simulink model "Simulation_parfait"  (Simulink 6.0)
settings: Solver=ode3  StartTime=0.0  StopTime=10  FixedStep=5e-4  RelTol=5e-3
undefined symbols (not defined in the file or in its folder): sigbuilder_block
libraries: simulink x23, mblibv1 x15, aerolibtransform2 x5, vrlib x1
settings Model: LastModifiedBy=Yann
settings OptimizationCC: InlineInvariantSignals=off
settings SimMechanicsCC: VisDuringSimulation=on

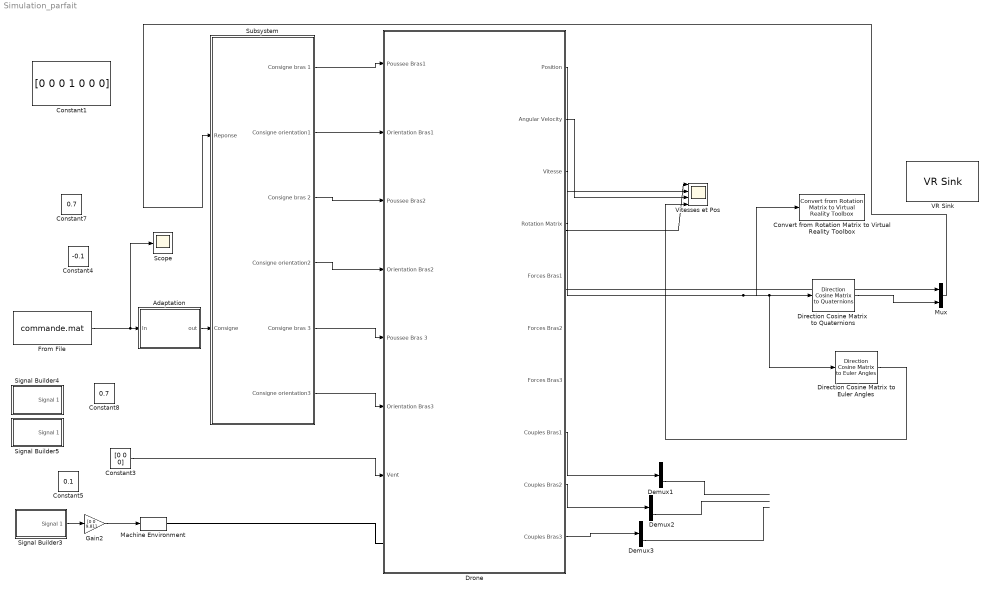
== system Simulation_parfait ==
  Adaptation : Subsystem
  Constant1 : Constant  Value=[0 0 0 1 0 0 0]
  Constant3 : Constant  Value=[0 0 0]
  Constant4 : Constant  Value=-0.1
  Constant5 : Constant  Value=0.1
  Constant7 : Constant  Value=0.7
  Constant8 : Constant  Value=0.7
  Convert from Rotation Matrix to Virtual Reality Toolbox : mblibv1/Utilities/Convert from Rotation Matrix to Virtual Reality Toolbox  Tag=Pose2VR
  Demux1 : Demux  Outputs=3
  Demux2 : Demux  Outputs=3
  Demux3 : Demux  Outputs=3
  Direction Cosine Matrix  to Quaternions : aerolibtransform2/Direction Cosine Matrix  to Quaternions
  Direction Cosine Matrix to Euler Angles : aerolibtransform2/Direction Cosine Matrix to Euler Angles
  Drone : Subsystem
  From File : FromFile  FileName=commande.mat  SampleTime=0
  Gain2 : Gain  Gain=[0 0 9.81]
  Machine Environment : mblibv1/Bodies/Machine Environment  Tag=Factory ground  DialogController=MECH.DialogSource  Opaque=on  PortType=env  PhysicalDomain=Mechanical  DialogTemplateClass=MECH.MachineEnvironment  SyncWhenCopied=off  Gravity=[0 0 9.81]  GravityUnits=m/s^2  GravityAsSignal=on  Dimensionality=Auto-detect  AnalysisType=Forward dynamics  LinearAssemblyTolerance=1e-3  LinearAssemblyToleranceUnits=m  AngularAssemblyTolerance=1e-3  AngularAssemblyToleranceUnits=rad  ConstraintSolverType=Stabilizing  ConstraintRelTolerance=1e-4  ConstraintAbsTolerance=1e-4  UseRobustSingularityHandling=off  StatePerturbationType=Fixed  PerturbationSize=1e-5  VisualizeMachine=on
  Mux : Mux  Inputs=2
  Scope : Scope
      settings: YMin=0  YMax=1  SaveName=ScopeData3
  Signal Builder3 : Subsystem  Tag=STV Subsys  LoadFcn=sigbuilder_block('load');  StartFcn=sigbuilder_block('start');  StopFcn=sigbuilder_block('stop');  ClipboardFcn=sigbuilder_block('clipboard');  mask(Sigbuilder block){}
      mask help: Sigbuilder GUI
      mask init:
      | if ~strcmp(get_param(bdroot(gcbh),'SimulationStatus'),'stopped') tuvar = sigbuilder_block('maskInit'); end
      settings: CopyFcn=sigbuilder_block('copy');  DeleteFcn=sigbuilder_block('delete');  ModelCloseFcn=sigbuilder_block('modelClose');  PreSaveFcn=sigbuilder_block('preSave');  NameChangeFcn=sigbuilder_block('namechange');  OpenFcn=sigbuilder_block('open',[39.75 63 664.5 410.25 ]);  CloseFcn=sigbuilder_block('close');
      mask Display: plot(0,0,100,100,[10,10,40,40,10],[80,20,20,80,80],[40,10],[50,50], [40,27,10],[65,72,56],[40,25,25,10],[28,28,43,43]);
  Signal Builder4 : Subsystem  Tag=STV Subsys  LoadFcn=sigbuilder_block('load');  StartFcn=sigbuilder_block('start');  StopFcn=sigbuilder_block('stop');  ClipboardFcn=sigbuilder_block('clipboard');  mask(Sigbuilder block){}
      mask help: Sigbuilder GUI
      mask init:
      | if ~strcmp(get_param(bdroot(gcbh),'SimulationStatus'),'stopped') tuvar = sigbuilder_block('maskInit'); end
      settings: CopyFcn=sigbuilder_block('copy');  DeleteFcn=sigbuilder_block('delete');  ModelCloseFcn=sigbuilder_block('modelClose');  PreSaveFcn=sigbuilder_block('preSave');  NameChangeFcn=sigbuilder_block('namechange');  OpenFcn=sigbuilder_block('open',[39.75 63 664.5 410.25 ]);  CloseFcn=sigbuilder_block('close');
      mask Display: plot(0,0,100,100,[10,10,40,40,10],[80,20,20,80,80],[40,10],[50,50], [40,27,10],[65,72,56],[40,25,25,10],[28,28,43,43]);
  Signal Builder5 : Subsystem  Tag=STV Subsys  LoadFcn=sigbuilder_block('load');  StartFcn=sigbuilder_block('start');  StopFcn=sigbuilder_block('stop');  ClipboardFcn=sigbuilder_block('clipboard');  mask(Sigbuilder block){}
      mask help: Sigbuilder GUI
      mask init:
      | if ~strcmp(get_param(bdroot(gcbh),'SimulationStatus'),'stopped') tuvar = sigbuilder_block('maskInit'); end
      settings: CopyFcn=sigbuilder_block('copy');  DeleteFcn=sigbuilder_block('delete');  ModelCloseFcn=sigbuilder_block('modelClose');  PreSaveFcn=sigbuilder_block('preSave');  NameChangeFcn=sigbuilder_block('namechange');  OpenFcn=sigbuilder_block('open',[75 91.5 664.5 410.25 ]);  CloseFcn=sigbuilder_block('close');
      mask Display: plot(0,0,100,100,[10,10,40,40,10],[80,20,20,80,80],[40,10],[50,50], [40,27,10],[65,72,56],[40,25,25,10],[28,28,43,43]);
  Subsystem : Subsystem
  VR Sink : vrlib/VR Sink  SampleTime=0.1  ViewEnable=on  RemoteChange=off  RemoteView=on  FieldsWritten=Drone.center.3.1.double#Drone.rotation.4.1.double  WorldFileName=drone2.WRL  AutoView=off  FigureProperties={}
  Vitesses et Pos : Scope  NumInputPorts=4
      settings: YMin=-0.15~-0.5~-9000~-5  YMax=0.25~0.9~4000~5  SaveName=ScopeData4
  wires:
  Drone/1(Position) -> Vitesses et Pos/1, Mux/1
  Drone/3(Vitesse) -> Vitesses et Pos/2
  Drone/2(Angular Velocity) -> Vitesses et Pos/3
  Drone/4(Rotation Matrix) -> Convert from Rotation Matrix to Virtual Reality Toolbox/1, Direction Cosine Matrix  to Quaternions/1, Direction Cosine Matrix to Euler Angles/1
  Constant3/1 -> Drone/7(Vent)
  Demux1/3 -> ?
  Demux2/3 -> ?
  Demux3/3 -> ?
  Drone/8(Couples Bras1) -> Demux1/1
  Drone/9(Couples Bras2) -> Demux2/1
  Drone/10(Couples Bras3) -> Demux3/1
  Signal Builder3/1(Signal 1) -> Gain2/1
  Gain2/1 -> Machine Environment/1
  Direction Cosine Matrix  to Quaternions/1 -> Mux/2
  Mux/1 -> Subsystem/1(Reponse)
  From File/1 -> Scope/1, Adaptation/1(In)
  Subsystem/1(Consigne bras 1) -> Drone/1(Poussee Bras1)
  Subsystem/5(Consigne bras 3) -> Drone/5(Poussee Bras 3)
  Subsystem/6(Consigne orientation3) -> Drone/6(Orientation Bras3)
  Direction Cosine Matrix to Euler Angles/1 -> Vitesses et Pos/4
  Subsystem/4(Consigne orientation2) -> Drone/4(Orientation Bras2)
  Subsystem/3(Consigne bras 2) -> Drone/3(Poussee Bras2)
  Subsystem/2(Consigne orientation1) -> Drone/2(Orientation Bras1)
  Adaptation/1(out) -> Subsystem/2(Consigne)
  connections:
  Drone/LConn1 -- Machine Environment/RConn1

== system Simulation_parfait/Adaptation ==
  In : Inport  Port=1  LatchInput=off
  Demux : Demux  Outputs=2
  Euler Angles to Quaternions : aerolibtransform2/Euler Angles to Quaternions
  Mux : Mux  Inputs=2
  Reshape : simulink/Math Operations/Reshape  OutputDimensionality=1-D array  OutputDimensions=[1,1]
  out : Outport
  wires:
  In/1 -> Demux/1
  Demux/2 -> Euler Angles to Quaternions/1
  Euler Angles to Quaternions/1 -> Mux/2
  Demux/1 -> Mux/1
  Mux/1 -> Reshape/1
  Reshape/1 -> out/1

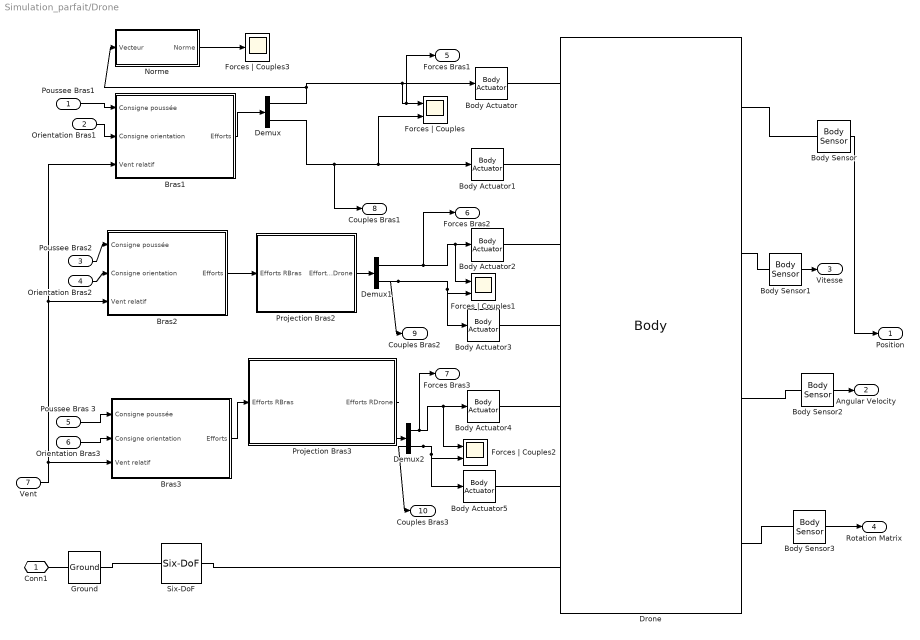
== system Simulation_parfait/Drone ==
  Poussee Bras1 : Inport  Port=1  LatchInput=off
  Orientation Bras1 : Inport  Port=2  LatchInput=off
  Poussee Bras2 : Inport  Port=3  LatchInput=off
  Orientation Bras2 : Inport  Port=4  LatchInput=off
  Poussee Bras 3 : Inport  Port=5  LatchInput=off
  Orientation Bras3 : Inport  Port=6  LatchInput=off
  Vent : Inport  Port=7  LatchInput=off
  Body Actuator : mblibv1/Sensors &  Actuators/Body Actuator  Opaque=on  PhysicalDomain=Mechanical  PortType=blob  ActuationStyle=Force  AngleUnits=deg  ArcVelocityUnits=deg/s  ArcAccelerationUnits=deg/s^2  CoordPositionUnits=m  VelocityUnits=m/s  AccelerationUnits=m/s^2  ForceUnits=N  TorqueUnits=N-m  ActiveIO=on  Width=3  DialogClass=MechanicalActuatorBlock  ReferenceFrame=Local (Body CS)  Angle=off  CoordPosition=on  Force=on  Torque=off
  Body Actuator1 : mblibv1/Sensors &  Actuators/Body Actuator  Opaque=on  PhysicalDomain=Mechanical  PortType=blob  ActuationStyle=Force  AngleUnits=deg  ArcVelocityUnits=deg/s  ArcAccelerationUnits=deg/s^2  CoordPositionUnits=m  VelocityUnits=m/s  AccelerationUnits=m/s^2  ForceUnits=N  TorqueUnits=N-m  ActiveIO=on  Width=3  DialogClass=MechanicalActuatorBlock  ReferenceFrame=Local (Body CS)  Angle=off  CoordPosition=on  Force=off  Torque=on
  Body Actuator2 : mblibv1/Sensors &  Actuators/Body Actuator  Opaque=on  PhysicalDomain=Mechanical  PortType=blob  ActuationStyle=Force  AngleUnits=deg  ArcVelocityUnits=deg/s  ArcAccelerationUnits=deg/s^2  CoordPositionUnits=m  VelocityUnits=m/s  AccelerationUnits=m/s^2  ForceUnits=N  TorqueUnits=N-m  ActiveIO=on  Width=3  DialogClass=MechanicalActuatorBlock  ReferenceFrame=Local (Body CS)  Angle=off  CoordPosition=on  Force=on  Torque=off
  Body Actuator3 : mblibv1/Sensors &  Actuators/Body Actuator  Opaque=on  PhysicalDomain=Mechanical  PortType=blob  ActuationStyle=Force  AngleUnits=deg  ArcVelocityUnits=deg/s  ArcAccelerationUnits=deg/s^2  CoordPositionUnits=m  VelocityUnits=m/s  AccelerationUnits=m/s^2  ForceUnits=N  TorqueUnits=N-m  ActiveIO=on  Width=3  DialogClass=MechanicalActuatorBlock  ReferenceFrame=Local (Body CS)  Angle=off  CoordPosition=on  Force=off  Torque=on
  Body Actuator4 : mblibv1/Sensors &  Actuators/Body Actuator  Opaque=on  PhysicalDomain=Mechanical  PortType=blob  ActuationStyle=Force  AngleUnits=deg  ArcVelocityUnits=deg/s  ArcAccelerationUnits=deg/s^2  CoordPositionUnits=m  VelocityUnits=m/s  AccelerationUnits=m/s^2  ForceUnits=N  TorqueUnits=N-m  ActiveIO=on  Width=3  DialogClass=MechanicalActuatorBlock  ReferenceFrame=Local (Body CS)  Angle=off  CoordPosition=on  Force=on  Torque=off
  Body Actuator5 : mblibv1/Sensors &  Actuators/Body Actuator  Opaque=on  PhysicalDomain=Mechanical  PortType=blob  ActuationStyle=Force  AngleUnits=deg  ArcVelocityUnits=deg/s  ArcAccelerationUnits=deg/s^2  CoordPositionUnits=m  VelocityUnits=m/s  AccelerationUnits=m/s^2  ForceUnits=N  TorqueUnits=N-m  ActiveIO=on  Width=3  DialogClass=MechanicalActuatorBlock  ReferenceFrame=Local (Body CS)  Angle=off  CoordPosition=on  Force=off  Torque=on
  Body Sensor : mblibv1/Sensors &  Actuators/Body Sensor  Opaque=on  PhysicalDomain=Mechanical  PortType=blob  Muxed=on  Pose=off  Angle=on  AngleUnits=deg  ArcVelocity=off  ArcVelocityUnits=deg/s  ArcAcceleration=off  ArcAccelerationUnits=deg/s^2  CoordPosition=on  CoordPositionUnits=m  Velocity=off  VelocityUnits=m/s  Acceleration=off  AccelerationUnits=m/s^2  Quaternion=on  QuaternionDT=off  QuaternionDDT=off  QuaternionUnits=off  OutputVector=[ 3 ]  ActiveIO=on  Width=3  DialogClass=MechanicalSensorBlock  ReferenceFrame=Absolute (World)
  Body Sensor1 : mblibv1/Sensors &  Actuators/Body Sensor  Opaque=on  PhysicalDomain=Mechanical  PortType=blob  Muxed=on  Pose=off  Angle=on  AngleUnits=deg  ArcVelocity=off  ArcVelocityUnits=deg/s  ArcAcceleration=off  ArcAccelerationUnits=deg/s^2  CoordPosition=off  CoordPositionUnits=m  Velocity=on  VelocityUnits=m/s  Acceleration=off  AccelerationUnits=m/s^2  Quaternion=on  QuaternionDT=off  QuaternionDDT=off  QuaternionUnits=off  OutputVector=[ 3 ]  ActiveIO=on  Width=3  DialogClass=MechanicalSensorBlock  ReferenceFrame=Absolute (World)
  Body Sensor2 : mblibv1/Sensors &  Actuators/Body Sensor  Opaque=on  PhysicalDomain=Mechanical  PortType=blob  Muxed=on  Pose=off  Angle=on  AngleUnits=deg  ArcVelocity=on  ArcVelocityUnits=deg/s  ArcAcceleration=off  ArcAccelerationUnits=deg/s^2  CoordPosition=off  CoordPositionUnits=m  Velocity=off  VelocityUnits=m/s  Acceleration=off  AccelerationUnits=m/s^2  Quaternion=on  QuaternionDT=off  QuaternionDDT=off  QuaternionUnits=off  OutputVector=[ 3 ]  ActiveIO=on  Width=3  DialogClass=MechanicalSensorBlock  ReferenceFrame=Absolute (World)
  Body Sensor3 : mblibv1/Sensors &  Actuators/Body Sensor  Opaque=on  PhysicalDomain=Mechanical  PortType=blob  Muxed=on  Pose=on  Angle=on  AngleUnits=deg  ArcVelocity=off  ArcVelocityUnits=deg/s  ArcAcceleration=off  ArcAccelerationUnits=deg/s^2  CoordPosition=off  CoordPositionUnits=m  Velocity=off  VelocityUnits=m/s  Acceleration=off  AccelerationUnits=m/s^2  Quaternion=on  QuaternionDT=off  QuaternionDDT=off  QuaternionUnits=off  OutputVector=[ 9 ]  ActiveIO=on  Width=9  DialogClass=MechanicalSensorBlock  ReferenceFrame=Absolute (World)
  Bras1 : Subsystem
  Bras2 : Subsystem
  Bras3 : Subsystem
  Demux : Demux  Outputs=2
  Demux1 : Demux  Outputs=2
  Demux2 : Demux  Outputs=2
  Drone : mblibv1/Bodies/Body  PhysicalDomain=mechanical  SubClassName=Unknown  LeftPortType=workingframe  RightPortType=workingframe  LConnTagsString=CS3|CS9|CS5|CS10|CS4|CS11|CS1  RConnTagsString=CS2|CS6|CS7|CS8  DialogClass=MechanicalBodyBlock  Mass=1.331  MassUnits=kg  InertiaUnits=kg*m^2  Inertia=[1e-2 9.762e-8 1.027e-6;9.762e-8 0.01 -6.855e-6; 1.027e-6 -6.855e-6 0.018 ]  Shape=Cylinder  ShapeDims=[1 1]  ShapeUnits=m  ShapeUse=false  Density=1  DensityUnits=kg/m^3  DensityUse=false  CG=Left$CG$[0 0 0]$WORLD$WORLD$m$[0 0 0]$Euler X-Y-Z$deg$WORLD$false  WorkingFrames=Right$CS2$[0 0 0]$CG$CG$m$[0 0 0]$Euler X-Y-Z$deg$WORLD$true#Left$CS3$[0.21 0 0]$CG$CG$m$[0 0 0]$Euler X-Y-Z$deg$WORLD$true#Left$CS9$[0.21 0 0]$CG$CG$m$[0 0 0]$Euler X-Y-Z$deg$WORLD$true#Left$CS5$[-0.105 0.1819 0]$CG$CG$m$[0 0 0]$Euler X-Y-Z$deg$WORLD$true#Left$CS10$[-0.105 0.1819 0]$CG$CG$m$[0 0 0]$Euler X-Y-Z$deg$WORLD$true#Left$CS4$[-0.105 -0.1819 0]$CG$CG$m$[0 0 0]$Euler X-Y-Z$deg$WORLD$true#Left$CS11$[-0.105 -0.1819 0]$CG$CG$m$[0 0 0]$Euler X-Y-Z$deg$WORLD$true#Right$CS6$[0 0 0]$CG$CG$m$[0 0 0]$Euler X-Y-Z$deg$WORLD$true#Right$CS7$[0 0 0]$CG$CG$m$[0 0 0]$Euler X-Y-Z$deg$WORLD$true#Right$CS8$[0 0 0]$CG$CG$m$[0 0 0]$Euler X-Y-Z$deg$WORLD$true#Left$CS1$[0 0 0]$CG$CG$m$[0 0 0]$Euler X-Y-Z$deg$WORLD$true#Right$CS12$[0 0 0]$CG$CG$m$[0 0 0]$Euler X-Y-Z$deg$WORLD$false
  Forces | Couples : Scope  NumInputPorts=2
      settings: YMin=-0.025~-1.5  YMax=0.04~0
  Forces | Couples1 : Scope  NumInputPorts=2
      settings: YMin=-4~-1.25  YMax=0.5~0
  Forces | Couples2 : Scope  NumInputPorts=2
      settings: YMin=-6~-1.5  YMax=1~1.25  SaveName=ScopeData2
  Forces | Couples3 : Scope
      settings: YMin=0  YMax=5.5  SaveName=ScopeData16
  Ground : mblibv1/Bodies/Ground  Opaque=on  LeftPortType=env  RightPortType=workingframe  PhysicalDomain=Mechanical  DialogClass=GroundBlock  CoordPosition=[0 0 0]  CoordPositionUnits=m  StateVectorMgrId=-1  MachineId=[1 0]  ShowEnvPort=on
  Norme : Subsystem  mask{ordre=2}
      mask Display: text(0.3,0.5,strcat('Norme',get_param(gcb, 'ordre')));
  Projection Bras2 : Subsystem
  Projection Bras3 : Subsystem
  Six-DoF : mblibv1/Joints/Six-DoF  PhysicalDomain=mechanical  SubClassName=Unknown  LeftPortType=blob  RightPortType=blob  LConnTagsString=__newl0  RConnTagsString=__newr0  NumSAPorts=0  CutJoint=off  MarkAsCut=off  Primitives=prismatic_prismatic_prismatic_spherical  PrimitiveProps=P1$INERTIAL$[1 0 0]$prismatic#P2$INERTIAL$[0 1 0]$prismatic#P3$INERTIAL$[0 0 1]$prismatic#S$INERTIAL$[0 0 0]$spherical  DialogClass=JointBlock
  Conn1 : PMIOPort  Port=1  Side=Left
  Position : Outport
  Angular Velocity : Outport  Port=2
  Vitesse : Outport  Port=3
  Rotation Matrix : Outport  Port=4
  Forces Bras1 : Outport  Port=5
  Forces Bras2 : Outport  Port=6
  Forces Bras3 : Outport  Port=7
  Couples Bras1 : Outport  Port=8
  Couples Bras2 : Outport  Port=9
  Couples Bras3 : Outport  Port=10
  wires:
  Body Sensor/1 -> Position/1
  Body Sensor2/1 -> Angular Velocity/1
  Body Sensor1/1 -> Vitesse/1
  Body Sensor3/1 -> Rotation Matrix/1
  Vent/1 -> Bras1/3(Vent relatif), Bras2/3(Vent relatif), Bras3/3(Vent relatif)
  Poussee Bras 3/1 -> Bras3/1(Consigne poussée)
  Orientation Bras2/1 -> Bras2/2(Consigne orientation)
  Orientation Bras3/1 -> Bras3/2(Consigne orientation)
  Orientation Bras1/1 -> Bras1/2(Consigne orientation)
  Poussee Bras1/1 -> Bras1/1(Consigne poussée)
  Poussee Bras2/1 -> Bras2/1(Consigne poussée)
  Demux1/1 -> Body Actuator2/1, Forces | Couples1/1, Forces Bras2/1
  Demux1/2 -> Body Actuator3/1, Forces | Couples1/2, Couples Bras2/1
  Projection Bras2/1(Efforts RDrone) -> Demux1/1
  Demux2/1 -> Body Actuator4/1, Forces | Couples2/1, Forces Bras3/1
  Demux2/2 -> Body Actuator5/1, Forces | Couples2/2, Couples Bras3/1
  Projection Bras3/1(Efforts RDrone) -> Demux2/1
  Bras1/1(Efforts) -> Demux/1
  Demux/1 -> Body Actuator/1, Forces | Couples/1, Forces Bras1/1, Norme/1(Vecteur)
  Demux/2 -> Body Actuator1/1, Forces | Couples/2, Couples Bras1/1
  Norme/1(Norme) -> Forces | Couples3/1
  Bras2/1(Efforts) -> Projection Bras2/1(Efforts RBras)
  Bras3/1(Efforts) -> Projection Bras3/1(Efforts RBras)
  connections:
  Body Actuator/RConn1 -- Drone/LConn1
  Body Actuator1/RConn1 -- Drone/LConn2
  Body Actuator2/RConn1 -- Drone/LConn3
  Body Actuator3/RConn1 -- Drone/LConn4
  Body Actuator4/RConn1 -- Drone/LConn5
  Body Actuator5/RConn1 -- Drone/LConn6
  Body Sensor/LConn1 -- Drone/RConn1
  Body Sensor1/LConn1 -- Drone/RConn2
  Drone/RConn3 -- Body Sensor2/LConn1
  Body Sensor3/LConn1 -- Drone/RConn4
  Six-DoF/RConn1 -- Drone/LConn7
  Ground/RConn1 -- Six-DoF/LConn1
  Conn1/RConn1 -- Ground/LConn1

== system Simulation_parfait/Signal Builder3 ==
  Demux : Demux  Tag=STV Demux  Outputs=1
  FromWs : FromWorkspace  Tag=STV FromWs  VariableName=tuvar  SampleTime=0  SigBuilderData=DataTag1  VnvData=DataTag2
      SigBuilderData=|
      | channels.label = 'Signal 1'
      | channels.allXData = {[0 10]}
      | channels.allYData = {[1 1]}
      | common.afterFinalStr = 'Extrapolate'
      | common.sampleTime = 0
      | dataSet.timeRange = [0 10]
      | dataSet.name = 'Group 1'
  Signal 1 : Outport  Tag=STV Outport
  wires:
  Demux/1 -> Signal 1/1
  FromWs/1 -> Demux/1

== system Simulation_parfait/Signal Builder4 ==
  Demux : Demux  Tag=STV Demux  Outputs=1
  FromWs : FromWorkspace  Tag=STV FromWs  VariableName=tuvar  SampleTime=0  SigBuilderData=DataTag3  VnvData=DataTag4
      SigBuilderData=|
      | channels.label = 'Signal 1'
      | channels.allXData = {[0 1.02 1.1 2.46 2.54 3.88 4.08 10]}
      | channels.allYData = {[0 0 1 1.005 0.005 0.0041018766756 0.805 0.8]}
      | common.afterFinalStr = 'Extrapolate'
      | common.sampleTime = 0
      | dataSet.timeRange = [0 10]
      | dataSet.name = 'Group 1'
  Signal 1 : Outport  Tag=STV Outport
  wires:
  Demux/1 -> Signal 1/1
  FromWs/1 -> Demux/1

== system Simulation_parfait/Signal Builder5 ==
  Demux : Demux  Tag=STV Demux  Outputs=1
  FromWs : FromWorkspace  Tag=STV FromWs  VariableName=tuvar  SampleTime=0  SigBuilderData=DataTag5  VnvData=DataTag6
      SigBuilderData=|
      | channels.label = 'Signal 1'
      | channels.allXData = {[0 5.92 6.1 7.4 7.78 8.78 8.94 10]}
      | channels.allYData = {[0 0 0.5 0.49 -0.4 -0.4 0 0]}
      | common.afterFinalStr = 'Extrapolate'
      | common.sampleTime = 0
      | dataSet.timeRange = [0 10]
      | dataSet.name = 'Group 1'
  Signal 1 : Outport  Tag=STV Outport
  wires:
  Demux/1 -> Signal 1/1
  FromWs/1 -> Demux/1

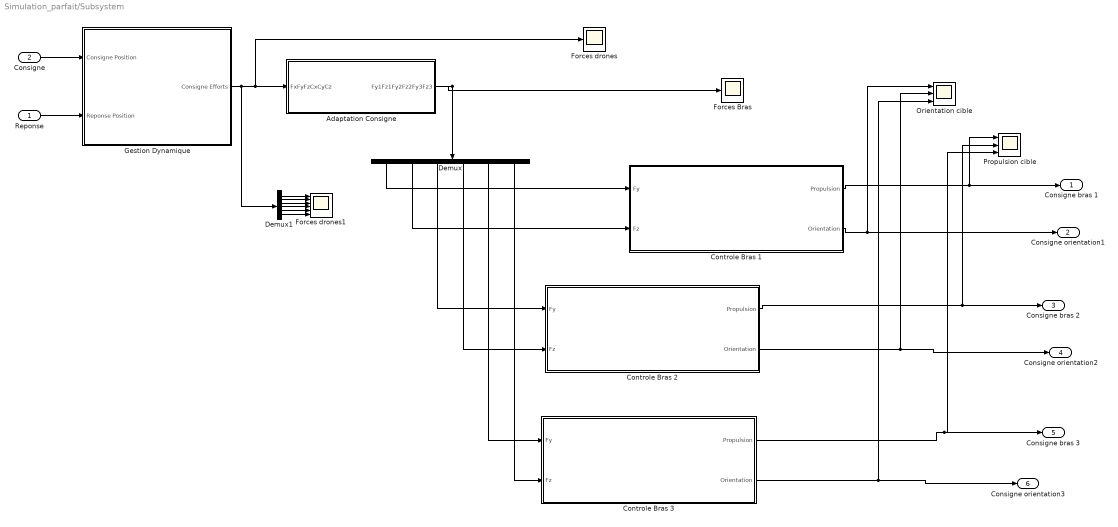
== system Simulation_parfait/Subsystem ==
  Reponse : Inport  Port=1  LatchInput=off
  Consigne : Inport  Port=2  LatchInput=off
  Adaptation Consigne : Subsystem  mask{l=0.21}
      mask prompts: l "Longueur Bras"
  Controle Bras 1 : Subsystem
  Controle Bras 2 : Subsystem
  Controle Bras 3 : Subsystem
  Demux : Demux  Orientation=down  Outputs=6
  Demux1 : Demux  Outputs=6
  Forces Bras : Scope
      settings: YMin=-0.24  YMax=2.77556e-017  SaveName=ScopeData14
  Forces drones : Scope
      settings: YMin=-0.01  YMax=0.0005  SaveName=ScopeData5
  Forces drones1 : Scope  NumInputPorts=6
      settings: YMin=-0.01~-5~-5~-5~-5~-5  YMax=0.0005~5~5~5~5~5  SaveName=ScopeData12
  Gestion Dynamique : Subsystem
  Orientation cible : Scope  NumInputPorts=3
      settings: YMin=-3.5~-5~-5  YMax=3.5~5~5  SaveName=ScopeData15
  Propulsion cible : Scope  NumInputPorts=3
      settings: YMin=1.9~0~-5  YMax=2.1~2~5  SaveName=ScopeData9
  Consigne bras 1 : Outport
  Consigne orientation1 : Outport  Port=2
  Consigne bras 2 : Outport  Port=3
  Consigne orientation2 : Outport  Port=4
  Consigne bras 3 : Outport  Port=5
  Consigne orientation3 : Outport  Port=6
  wires:
  Gestion Dynamique/1(Consigne Efforts) -> Adaptation Consigne/1(FxFyFzCxCyCz), Forces drones/1, Demux1/1
  Reponse/1 -> Gestion Dynamique/2(Reponse Position)
  Consigne/1 -> Gestion Dynamique/1(Consigne Position)
  Demux/1 -> Controle Bras 1/1(Fy)
  Demux/2 -> Controle Bras 1/2(Fz)
  Adaptation Consigne/1(Fy1Fz1Fy2Fz2Fy3Fz3) -> Demux/1, Forces Bras/1
  Demux/3 -> Controle Bras 2/1(Fy)
  Demux/4 -> Controle Bras 2/2(Fz)
  Demux/5 -> Controle Bras 3/1(Fy)
  Demux/6 -> Controle Bras 3/2(Fz)
  Controle Bras 1/1(Propulsion) -> Consigne bras 1/1, Propulsion cible/1
  Controle Bras 1/2(Orientation) -> Consigne orientation1/1, Orientation cible/1
  Controle Bras 2/1(Propulsion) -> Consigne bras 2/1, Propulsion cible/2
  Controle Bras 2/2(Orientation) -> Consigne orientation2/1, Orientation cible/2
  Controle Bras 3/1(Propulsion) -> Consigne bras 3/1, Propulsion cible/3
  Controle Bras 3/2(Orientation) -> Consigne orientation3/1, Orientation cible/3
  Demux1/1 -> Forces drones1/1
  Demux1/2 -> Forces drones1/2
  Demux1/3 -> Forces drones1/3
  Demux1/4 -> Forces drones1/4
  Demux1/5 -> Forces drones1/5
  Demux1/6 -> Forces drones1/6

== system Simulation_parfait/Drone/Bras1 ==
  Consigne poussée : Inport  Port=1  LatchInput=off
  Consigne orientation : Inport  Port=2  LatchInput=off
  Vent relatif : Inport  Port=3  LatchInput=off
  Bus Creator : BusCreator  DialogController=Simulink.DDGSource_Bus  Inputs=2
  Constant : Constant  Value=[0 0 0]
  Gain : Gain  Gain=pi
  Matrice rotation force : Subsystem
  Terminator : Terminator
  Efforts : Outport
  wires:
  Matrice rotation force/1(Force) -> Bus Creator/1  "Resultante"
  Constant/1 -> Bus Creator/2  "Moments"
  Bus Creator/1 -> Efforts/1
  Consigne orientation/1 -> Gain/1
  Consigne poussée/1 -> Matrice rotation force/1(Force poussée)
  Gain/1 -> Matrice rotation force/2(Angle orientation)
  Vent relatif/1 -> Terminator/1

== system Simulation_parfait/Drone/Bras2 ==
  Consigne poussée : Inport  Port=1  LatchInput=off
  Consigne orientation : Inport  Port=2  LatchInput=off
  Vent relatif : Inport  Port=3  LatchInput=off
  Bus Creator : BusCreator  DialogController=Simulink.DDGSource_Bus  Inputs=2
  Constant : Constant  Value=[0 0 0]
  Gain : Gain  Gain=pi
  Matrice rotation force : Subsystem
  Terminator : Terminator
  Efforts : Outport
  wires:
  Matrice rotation force/1(Force) -> Bus Creator/1  "Resultante"
  Constant/1 -> Bus Creator/2  "Moments"
  Bus Creator/1 -> Efforts/1
  Consigne orientation/1 -> Gain/1
  Consigne poussée/1 -> Matrice rotation force/1(Force poussée)
  Gain/1 -> Matrice rotation force/2(Angle orientation)
  Vent relatif/1 -> Terminator/1

== system Simulation_parfait/Drone/Bras3 ==
  Consigne poussée : Inport  Port=1  LatchInput=off
  Consigne orientation : Inport  Port=2  LatchInput=off
  Vent relatif : Inport  Port=3  LatchInput=off
  Bus Creator : BusCreator  DialogController=Simulink.DDGSource_Bus  Inputs=2
  Constant : Constant  Value=[0 0 0]
  Gain : Gain  Gain=pi
  Matrice rotation force : Subsystem
  Terminator : Terminator
  Efforts : Outport
  wires:
  Matrice rotation force/1(Force) -> Bus Creator/1  "Resultante"
  Constant/1 -> Bus Creator/2  "Moments"
  Bus Creator/1 -> Efforts/1
  Consigne orientation/1 -> Gain/1
  Consigne poussée/1 -> Matrice rotation force/1(Force poussée)
  Gain/1 -> Matrice rotation force/2(Angle orientation)
  Vent relatif/1 -> Terminator/1

== system Simulation_parfait/Drone/Norme ==
  Vecteur : Inport  Port=1  LatchInput=off
  Constant1 : Constant  Value=ordre
  Math Function : Math  Operator=pow  SaturateOnIntegerOverflow=on
  Math Function1 : Math  Operator=reciprocal  SaturateOnIntegerOverflow=on
  Math Function2 : Math  Operator=pow  SaturateOnIntegerOverflow=on
  Sum of Elements : Sum  Inputs=+  OutScaling=2^-10
  Norme : Outport
  wires:
  Math Function/1 -> Sum of Elements/1
  Vecteur/1 -> Math Function/1
  Constant1/1 -> Math Function/2, Math Function1/1
  Math Function1/1 -> Math Function2/2
  Sum of Elements/1 -> Math Function2/1
  Math Function2/1 -> Norme/1

== system Simulation_parfait/Drone/Projection Bras2 ==
  note: Forces
  note: Moments
  Efforts RBras : Inport  Port=1  LatchInput=off
  Bus Creator : BusCreator  DialogController=Simulink.DDGSource_Bus  Inputs=2
  Demux : Demux  Outputs=2
  Gain : Gain  Gain=[cos(2*pi/3) -sin(2*pi/3) 0 ; sin(2*pi/3) cos(2*pi/3) 0; 0 0 1]  Multiplication=Matrix(K*u) (u vector)
  Gain1 : Gain  Gain=[cos(2*pi/3) -sin(2*pi/3) 0 ; sin(2*pi/3) cos(2*pi/3) 0; 0 0 1]  Multiplication=Matrix(K*u) (u vector)
  Efforts RDrone : Outport
  wires:
  Efforts RBras/1 -> Demux/1
  Demux/1 -> Gain/1
  Demux/2 -> Gain1/1
  Bus Creator/1 -> Efforts RDrone/1
  Gain/1 -> Bus Creator/1
  Gain1/1 -> Bus Creator/2

== system Simulation_parfait/Drone/Projection Bras3 ==
  note: Forces
  note: Moments
  Efforts RBras : Inport  Port=1  LatchInput=off
  Bus Creator : BusCreator  DialogController=Simulink.DDGSource_Bus  Inputs=2
  Demux : Demux  Outputs=2
  Matrice de Rotation : Gain  Gain=[cos(4*pi/3) -sin(4*pi/3) 0 ; sin(4*pi/3) cos(4*pi/3) 0; 0 0 1]  Multiplication=Matrix(K*u) (u vector)
  "Matrice de rotation " : Gain  Gain=[cos(4*pi/3) -sin(4*pi/3) 0 ; sin(4*pi/3) cos(4*pi/3) 0; 0 0 1]  Multiplication=Matrix(K*u) (u vector)
  Efforts RDrone : Outport
  wires:
  Efforts RBras/1 -> Demux/1
  Demux/1 -> Matrice de Rotation/1
  Demux/2 -> "Matrice de rotation "/1
  Bus Creator/1 -> Efforts RDrone/1
  Matrice de Rotation/1 -> Bus Creator/1
  "Matrice de rotation "/1 -> Bus Creator/2

== system Simulation_parfait/Subsystem/Adaptation Consigne ==
  FxFyFzCxCyCz : Inport  Port=1  LatchInput=off
  Matrice Correction : Constant  Value=[1 1 1 1/l 1/l -1/l]
  Matrice Transformation : Constant  Value=(1/3)*[0 2 0 0 0 1; 0 0 1 0 2 0; -sqrt(3) -1 0 0 0 1; 0 0 1 -sqrt(3) -1 0; sqrt(3) -1 0 0 0 1; 0 0 1 sqrt(3) -1 0]  VectorParams1D=off
  Product : Product  Multiplication=Matrix(*)  RndMeth=Zero
  Product1 : Product  RndMeth=Zero
  Fy1Fz1Fy2Fz2Fy3Fz3 : Outport
  wires:
  Product/1 -> Fy1Fz1Fy2Fz2Fy3Fz3/1
  Matrice Transformation/1 -> Product/1
  Matrice Correction/1 -> Product1/2
  FxFyFzCxCyCz/1 -> Product1/1
  Product1/1 -> Product/2

== system Simulation_parfait/Subsystem/Controle Bras 1 ==
  Fy : Inport  Port=1  LatchInput=off
  Fz : Inport  Port=2  LatchInput=off
  Adaptation Consigne1 : Subsystem  mask{a=2e-5, b=1e-3, c=2e-3}
  Controle Bras1 : Subsystem
  Gain : Gain  Gain=60/(500*2*pi)
  Gain5 : Gain  Gain=1/pi
  Propulsion : Outport
  Orientation : Outport  Port=2
  wires:
  Controle Bras1/1(Force Propulsion) -> Adaptation Consigne1/1(Force)
  Adaptation Consigne1/1(Consigne Omega) -> Gain/1
  Gain/1 -> Propulsion/1
  Fy/1 -> Controle Bras1/1(Fyc)
  Fz/1 -> Controle Bras1/2(Fzc)
  Gain5/1 -> Orientation/1
  Controle Bras1/2(Angle Orientation) -> Gain5/1

== system Simulation_parfait/Subsystem/Controle Bras 2 ==
  Fy : Inport  Port=1  LatchInput=off
  Fz : Inport  Port=2  LatchInput=off
  Adaptation Consigne1 : Subsystem  mask{a=2e-5, b=1e-3, c=2e-3}
  Controle Bras1 : Subsystem
  Gain : Gain  Gain=60/(500*2*pi)
  Gain5 : Gain  Gain=1/pi
  Propulsion : Outport
  Orientation : Outport  Port=2
  wires:
  Controle Bras1/1(Force Propulsion) -> Adaptation Consigne1/1(Force)
  Adaptation Consigne1/1(Consigne Omega) -> Gain/1
  Gain/1 -> Propulsion/1
  Fy/1 -> Controle Bras1/1(Fyc)
  Fz/1 -> Controle Bras1/2(Fzc)
  Gain5/1 -> Orientation/1
  Controle Bras1/2(Angle Orientation) -> Gain5/1

== system Simulation_parfait/Subsystem/Controle Bras 3 ==
  Fy : Inport  Port=1  LatchInput=off
  Fz : Inport  Port=2  LatchInput=off
  Adaptation Consigne1 : Subsystem  mask{a=2e-5, b=1e-3, c=2e-3}
  Controle Bras1 : Subsystem
  Gain : Gain  Gain=60/(500*2*pi)
  Gain5 : Gain  Gain=1/pi
  Propulsion : Outport
  Orientation : Outport  Port=2
  wires:
  Controle Bras1/1(Force Propulsion) -> Adaptation Consigne1/1(Force)
  Adaptation Consigne1/1(Consigne Omega) -> Gain/1
  Gain/1 -> Propulsion/1
  Fy/1 -> Controle Bras1/1(Fyc)
  Fz/1 -> Controle Bras1/2(Fzc)
  Gain5/1 -> Orientation/1
  Controle Bras1/2(Angle Orientation) -> Gain5/1

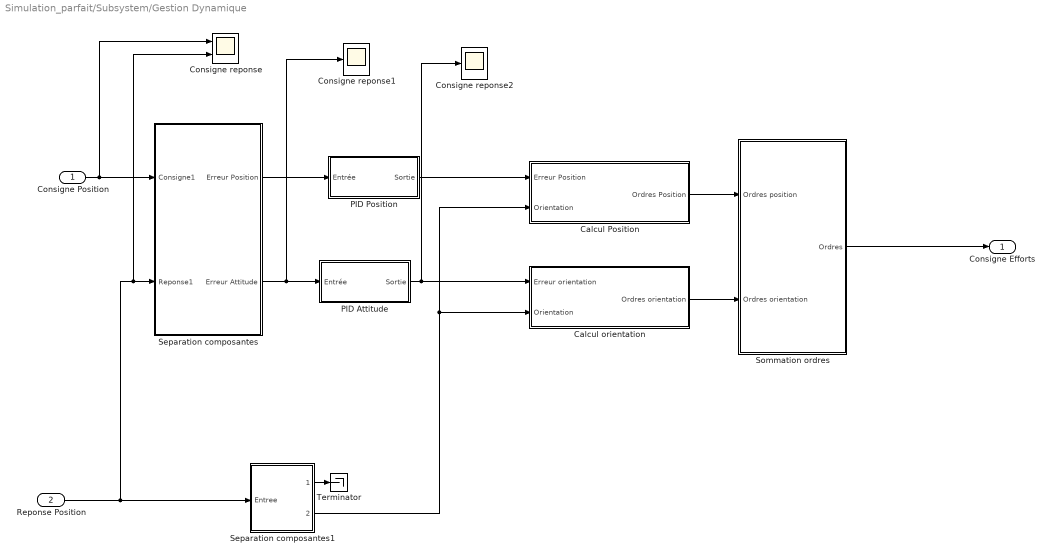
== system Simulation_parfait/Subsystem/Gestion Dynamique ==
  Consigne Position : Inport  Port=1  LatchInput=off
  Reponse Position : Inport  Port=2  LatchInput=off
  Calcul Position : Subsystem
  Calcul orientation : Subsystem
  Consigne reponse : Scope  NumInputPorts=2
      settings: YMin=0~-0.05  YMax=1~1.1  SaveName=ScopeData6
  Consigne reponse1 : Scope
      settings: YMin=0  YMax=1  SaveName=ScopeData8
  Consigne reponse2 : Scope
      settings: YMin=0  YMax=1  SaveName=ScopeData13
  PID Attitude : Subsystem  mask{kp=0.3, ki=0.1, kd=1, kdd=0}
  PID Position : Subsystem  mask{kp=100, ki=4, kd=1, kdd=0}
  Separation composantes : Subsystem
  Separation composantes1 : Subsystem
  Sommation ordres : Subsystem
  Terminator : Terminator
  Consigne Efforts : Outport
  wires:
  Reponse Position/1 -> Separation composantes1/1(Entree), Separation composantes/2(Reponse1), Consigne reponse/2
  Separation composantes1/2(Orientation) -> Calcul Position/2(Orientation), Calcul orientation/2(Orientation)
  Sommation ordres/1(Ordres) -> Consigne Efforts/1
  Separation composantes1/1(Position) -> Terminator/1
  PID Position/1(Sortie) -> Calcul Position/1(Erreur Position)
  Calcul Position/1(Ordres Position) -> Sommation ordres/1(Ordres position)
  Calcul orientation/1(Ordres orientation) -> Sommation ordres/2(Ordres orientation)
  PID Attitude/1(Sortie) -> Calcul orientation/1(Erreur orientation), Consigne reponse2/1
  Consigne Position/1 -> Separation composantes/1(Consigne1), Consigne reponse/1
  Separation composantes/1(Erreur Position) -> PID Position/1(Entrée)
  Separation composantes/2(Erreur Attitude) -> PID Attitude/1(Entrée), Consigne reponse1/1

== system Simulation_parfait/Drone/Bras1/Matrice rotation force ==
  Force poussée : Inport  Port=1  LatchInput=off
  Angle orientation : Inport  Port=2  LatchInput=off
  Constant : Constant  Value=0
  Cos : Trigonometry  Operator=cos
  Gain : Gain  Gain=[ 1 1 -1 ]
  Mux : Mux  Inputs=3
  Product : Product  RndMeth=Zero
  Reshape : simulink/Math Operations/Reshape  OutputDimensionality=1-D array  OutputDimensions=[1,1]
  Sin : Trigonometry
  Force : Outport
  wires:
  Angle orientation/1 -> Cos/1, Sin/1
  Constant/1 -> Mux/1
  Cos/1 -> Mux/3
  Sin/1 -> Mux/2
  Mux/1 -> Reshape/1
  Gain/1 -> Product/1
  Force poussée/1 -> Product/2
  Product/1 -> Force/1
  Reshape/1 -> Gain/1

== system Simulation_parfait/Drone/Bras2/Matrice rotation force ==
  Force poussée : Inport  Port=1  LatchInput=off
  Angle orientation : Inport  Port=2  LatchInput=off
  Constant : Constant  Value=0
  Cos : Trigonometry  Operator=cos
  Gain : Gain  Gain=[ 1 1 -1 ]
  Mux : Mux  Inputs=3
  Product : Product  RndMeth=Zero
  Reshape : simulink/Math Operations/Reshape  OutputDimensionality=1-D array  OutputDimensions=[1,1]
  Sin : Trigonometry
  Force : Outport
  wires:
  Angle orientation/1 -> Cos/1, Sin/1
  Constant/1 -> Mux/1
  Cos/1 -> Mux/3
  Sin/1 -> Mux/2
  Mux/1 -> Reshape/1
  Gain/1 -> Product/1
  Force poussée/1 -> Product/2
  Product/1 -> Force/1
  Reshape/1 -> Gain/1

== system Simulation_parfait/Drone/Bras3/Matrice rotation force ==
  Force poussée : Inport  Port=1  LatchInput=off
  Angle orientation : Inport  Port=2  LatchInput=off
  Constant : Constant  Value=0
  Cos : Trigonometry  Operator=cos
  Gain : Gain  Gain=[ 1 1 -1 ]
  Mux : Mux  Inputs=3
  Product : Product  RndMeth=Zero
  Reshape : simulink/Math Operations/Reshape  OutputDimensionality=1-D array  OutputDimensions=[1,1]
  Sin : Trigonometry
  Force : Outport
  wires:
  Angle orientation/1 -> Cos/1, Sin/1
  Constant/1 -> Mux/1
  Cos/1 -> Mux/3
  Sin/1 -> Mux/2
  Mux/1 -> Reshape/1
  Gain/1 -> Product/1
  Force poussée/1 -> Product/2
  Product/1 -> Force/1
  Reshape/1 -> Gain/1

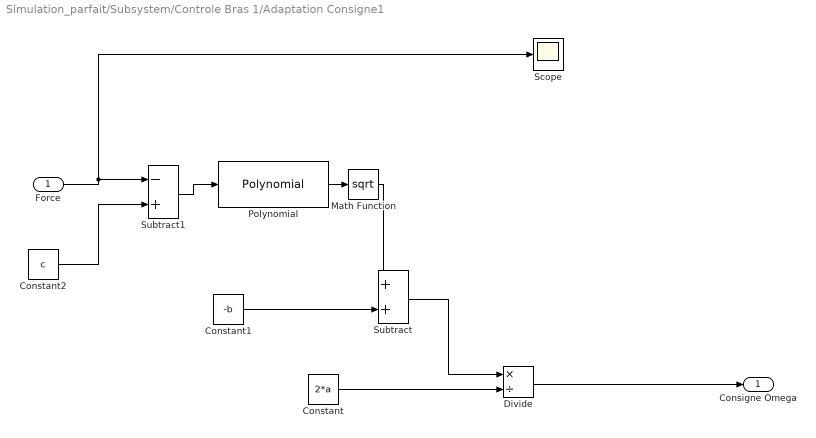
== system Simulation_parfait/Subsystem/Controle Bras 1/Adaptation Consigne1 ==
  Force : Inport  Port=1  LatchInput=off
  Constant : Constant  Value=2*a
  Constant1 : Constant  Value=-b
  Constant2 : Constant  Value=c
  Divide : Product  Inputs=*/  OutScaling=2^-10
  Math Function : Math  Operator=sqrt  SaturateOnIntegerOverflow=on
  Polynomial : simulink/Math Operations/Polynomial  coefs=[-4*a b*b]
  Scope : Scope
      settings: YMin=0  YMax=1000  SaveName=ScopeData7
  Subtract : Sum  OutScaling=2^-10
  Subtract1 : Sum  Inputs=-+  OutScaling=2^-10
  Consigne Omega : Outport
  wires:
  Constant/1 -> Divide/2
  Constant1/1 -> Subtract/2
  Subtract/1 -> Divide/1
  Divide/1 -> Consigne Omega/1
  Math Function/1 -> Subtract/1
  Polynomial/1 -> Math Function/1
  Force/1 -> Scope/1, Subtract1/1
  Subtract1/1 -> Polynomial/1
  Constant2/1 -> Subtract1/2

== system Simulation_parfait/Subsystem/Controle Bras 1/Controle Bras1 ==
  Fyc : Inport  Port=1  LatchInput=off
  Fzc : Inport  Port=2  LatchInput=off
  Complex to Magnitude-Angle : ComplexToMagnitudeAngle
  Real-Imag to Complex : RealImagToComplex
  Unary Minus : simulink/Math Operations/Unary Minus  DoSatur=off
  Force Propulsion : Outport
  Angle Orientation : Outport  Port=2
  wires:
  Real-Imag to Complex/1 -> Complex to Magnitude-Angle/1
  Complex to Magnitude-Angle/2 -> Angle Orientation/1
  Complex to Magnitude-Angle/1 -> Force Propulsion/1
  Fyc/1 -> Real-Imag to Complex/2
  Fzc/1 -> Unary Minus/1
  Unary Minus/1 -> Real-Imag to Complex/1

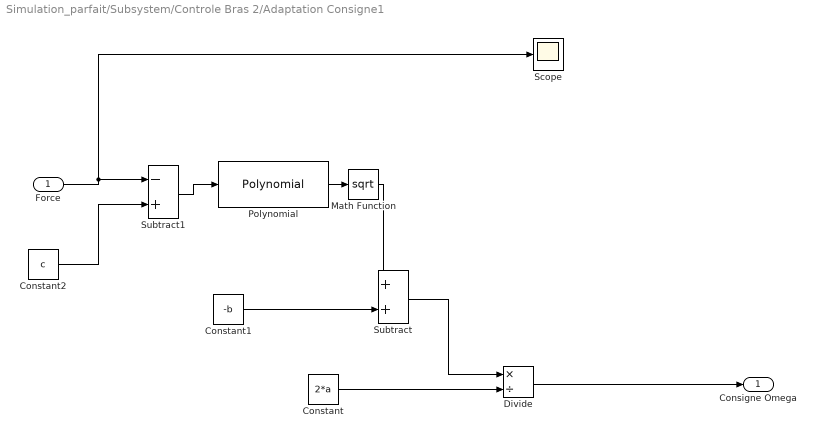
== system Simulation_parfait/Subsystem/Controle Bras 2/Adaptation Consigne1 ==
  Force : Inport  Port=1  LatchInput=off
  Constant : Constant  Value=2*a
  Constant1 : Constant  Value=-b
  Constant2 : Constant  Value=c
  Divide : Product  Inputs=*/  OutScaling=2^-10
  Math Function : Math  Operator=sqrt  SaturateOnIntegerOverflow=on
  Polynomial : simulink/Math Operations/Polynomial  coefs=[-4*a b*b]
  Scope : Scope
      settings: YMin=0  YMax=1000  SaveName=ScopeData7
  Subtract : Sum  OutScaling=2^-10
  Subtract1 : Sum  Inputs=-+  OutScaling=2^-10
  Consigne Omega : Outport
  wires:
  Constant/1 -> Divide/2
  Constant1/1 -> Subtract/2
  Subtract/1 -> Divide/1
  Divide/1 -> Consigne Omega/1
  Math Function/1 -> Subtract/1
  Polynomial/1 -> Math Function/1
  Force/1 -> Scope/1, Subtract1/1
  Subtract1/1 -> Polynomial/1
  Constant2/1 -> Subtract1/2

== system Simulation_parfait/Subsystem/Controle Bras 2/Controle Bras1 ==
  Fyc : Inport  Port=1  LatchInput=off
  Fzc : Inport  Port=2  LatchInput=off
  Complex to Magnitude-Angle : ComplexToMagnitudeAngle
  Real-Imag to Complex : RealImagToComplex
  Unary Minus : simulink/Math Operations/Unary Minus  DoSatur=off
  Force Propulsion : Outport
  Angle Orientation : Outport  Port=2
  wires:
  Real-Imag to Complex/1 -> Complex to Magnitude-Angle/1
  Complex to Magnitude-Angle/2 -> Angle Orientation/1
  Complex to Magnitude-Angle/1 -> Force Propulsion/1
  Fyc/1 -> Real-Imag to Complex/2
  Fzc/1 -> Unary Minus/1
  Unary Minus/1 -> Real-Imag to Complex/1

== system Simulation_parfait/Subsystem/Controle Bras 3/Adaptation Consigne1 ==
  Force : Inport  Port=1  LatchInput=off
  Constant : Constant  Value=2*a
  Constant1 : Constant  Value=-b
  Constant2 : Constant  Value=c
  Divide : Product  Inputs=*/  OutScaling=2^-10
  Math Function : Math  Operator=sqrt  SaturateOnIntegerOverflow=on
  Polynomial : simulink/Math Operations/Polynomial  coefs=[-4*a b*b]
  Scope : Scope
      settings: YMin=0  YMax=1000  SaveName=ScopeData7
  Subtract : Sum  OutScaling=2^-10
  Subtract1 : Sum  Inputs=-+  OutScaling=2^-10
  Consigne Omega : Outport
  wires:
  Constant/1 -> Divide/2
  Constant1/1 -> Subtract/2
  Subtract/1 -> Divide/1
  Divide/1 -> Consigne Omega/1
  Math Function/1 -> Subtract/1
  Polynomial/1 -> Math Function/1
  Force/1 -> Scope/1, Subtract1/1
  Subtract1/1 -> Polynomial/1
  Constant2/1 -> Subtract1/2

== system Simulation_parfait/Subsystem/Controle Bras 3/Controle Bras1 ==
  Fyc : Inport  Port=1  LatchInput=off
  Fzc : Inport  Port=2  LatchInput=off
  Complex to Magnitude-Angle : ComplexToMagnitudeAngle
  Real-Imag to Complex : RealImagToComplex
  Unary Minus : simulink/Math Operations/Unary Minus  DoSatur=off
  Force Propulsion : Outport
  Angle Orientation : Outport  Port=2
  wires:
  Real-Imag to Complex/1 -> Complex to Magnitude-Angle/1
  Complex to Magnitude-Angle/2 -> Angle Orientation/1
  Complex to Magnitude-Angle/1 -> Force Propulsion/1
  Fyc/1 -> Real-Imag to Complex/2
  Fzc/1 -> Unary Minus/1
  Unary Minus/1 -> Real-Imag to Complex/1

== system Simulation_parfait/Subsystem/Gestion Dynamique/Calcul Position ==
  Erreur Position : Inport  Port=1  LatchInput=off
  Orientation : Inport  Port=2  LatchInput=off
  Constant : Constant  Value=0
  Constant1 : Constant  Value=0
  Constant2 : Constant  Value=0
  Demux : Demux  Outputs=3
  Mux : Mux  Inputs=6
  Product : Product  Multiplication=Matrix(*)  RndMeth=Zero
  Quaternions to  Direction Cosine Matrix : aerolibtransform2/Quaternions to  Direction Cosine Matrix
  Reshape5 : simulink/Math Operations/Reshape  OutputDimensionality=1-D array  OutputDimensions=[1,1]
  Ordres Position : Outport
      settings: BusObject=perturbations
  wires:
  Mux/1 -> Reshape5/1
  Reshape5/1 -> Ordres Position/1
  Product/1 -> Demux/1
  Demux/1 -> Mux/1
  Demux/2 -> Mux/2
  Demux/3 -> Mux/3
  Constant2/1 -> Mux/6
  Constant1/1 -> Mux/5
  Constant/1 -> Mux/4
  Quaternions to  Direction Cosine Matrix/1 -> Product/1
  Orientation/1 -> Quaternions to  Direction Cosine Matrix/1
  Erreur Position/1 -> Product/2

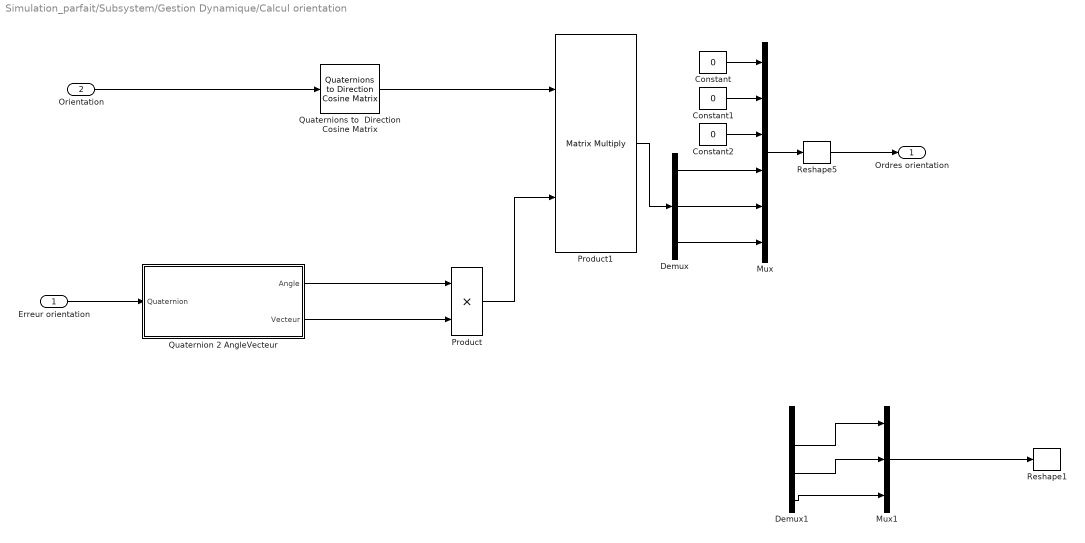
== system Simulation_parfait/Subsystem/Gestion Dynamique/Calcul orientation ==
  Erreur orientation : Inport  Port=1  LatchInput=off
  Orientation : Inport  Port=2  LatchInput=off
  Constant : Constant  Value=0
  Constant1 : Constant  Value=0
  Constant2 : Constant  Value=0
  Demux : Demux  Outputs=3
  Demux1 : Demux
  Mux : Mux  Inputs=6
  Mux1 : Mux  Inputs=3
  Product : Product  RndMeth=Zero
  Product1 : Product  Multiplication=Matrix(*)  RndMeth=Zero
  Quaternion 2 AngleVecteur : Subsystem
  Quaternions to  Direction Cosine Matrix : aerolibtransform2/Quaternions to  Direction Cosine Matrix
  Reshape1 : simulink/Math Operations/Reshape  OutputDimensionality=1-D array  OutputDimensions=[1,1]
  Reshape5 : simulink/Math Operations/Reshape  OutputDimensionality=1-D array  OutputDimensions=[1,1]
  Ordres orientation : Outport
      settings: BusObject=perturbations
  wires:
  Mux/1 -> Reshape5/1
  Reshape5/1 -> Ordres orientation/1
  Constant/1 -> Mux/1
  Constant1/1 -> Mux/2
  Constant2/1 -> Mux/3
  Demux/1 -> Mux/4
  Demux/2 -> Mux/5
  Demux/3 -> Mux/6
  Product1/1 -> Demux/1
  Orientation/1 -> Quaternions to  Direction Cosine Matrix/1
  Quaternion 2 AngleVecteur/2(Vecteur) -> Product/2
  Quaternion 2 AngleVecteur/1(Angle) -> Product/1
  Erreur orientation/1 -> Quaternion 2 AngleVecteur/1(Quaternion)
  Quaternions to  Direction Cosine Matrix/1 -> Product1/1
  Mux1/1 -> Reshape1/1
  Demux1/4 -> Mux1/3
  Demux1/3 -> Mux1/2
  Demux1/2 -> Mux1/1
  Product/1 -> Product1/2

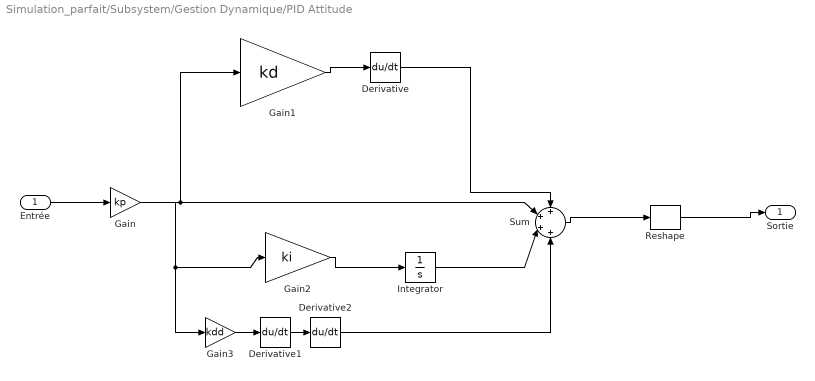
== system Simulation_parfait/Subsystem/Gestion Dynamique/PID Attitude ==
  Entrée : Inport  Port=1  LatchInput=off
  Derivative : Derivative
  Derivative1 : Derivative
  Derivative2 : Derivative
  Gain : Gain  Gain=kp
  Gain1 : Gain  Gain=kd
  Gain2 : Gain  Gain=ki
  Gain3 : Gain  Gain=kdd
  Integrator : Integrator
  Reshape : simulink/Math Operations/Reshape  OutputDimensionality=1-D array  OutputDimensions=[1,1]
  Sum : Sum  Inputs=++++
  Sortie : Outport
      settings: BusObject=perturbations
  wires:
  Entrée/1 -> Gain/1
  Gain/1 -> Sum/2, Gain1/1, Gain2/1, Gain3/1
  Derivative/1 -> Sum/1
  Integrator/1 -> Sum/3
  Gain2/1 -> Integrator/1
  Gain1/1 -> Derivative/1
  Sum/1 -> Reshape/1
  Gain3/1 -> Derivative1/1
  Derivative1/1 -> Derivative2/1
  Derivative2/1 -> Sum/4
  Reshape/1 -> Sortie/1

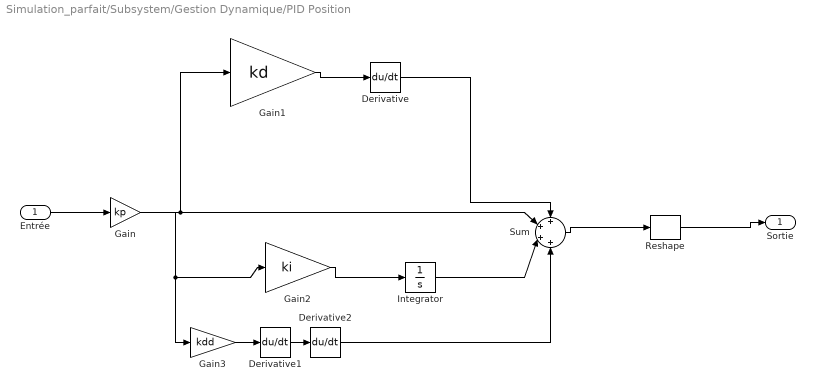
== system Simulation_parfait/Subsystem/Gestion Dynamique/PID Position ==
  Entrée : Inport  Port=1  LatchInput=off
  Derivative : Derivative
  Derivative1 : Derivative
  Derivative2 : Derivative
  Gain : Gain  Gain=kp
  Gain1 : Gain  Gain=kd
  Gain2 : Gain  Gain=ki
  Gain3 : Gain  Gain=kdd
  Integrator : Integrator
  Reshape : simulink/Math Operations/Reshape  OutputDimensionality=1-D array  OutputDimensions=[1,1]
  Sum : Sum  Inputs=++++
  Sortie : Outport
      settings: BusObject=perturbations
  wires:
  Entrée/1 -> Gain/1
  Gain/1 -> Sum/2, Gain1/1, Gain2/1, Gain3/1
  Derivative/1 -> Sum/1
  Integrator/1 -> Sum/3
  Gain2/1 -> Integrator/1
  Gain1/1 -> Derivative/1
  Sum/1 -> Reshape/1
  Gain3/1 -> Derivative1/1
  Derivative1/1 -> Derivative2/1
  Derivative2/1 -> Sum/4
  Reshape/1 -> Sortie/1

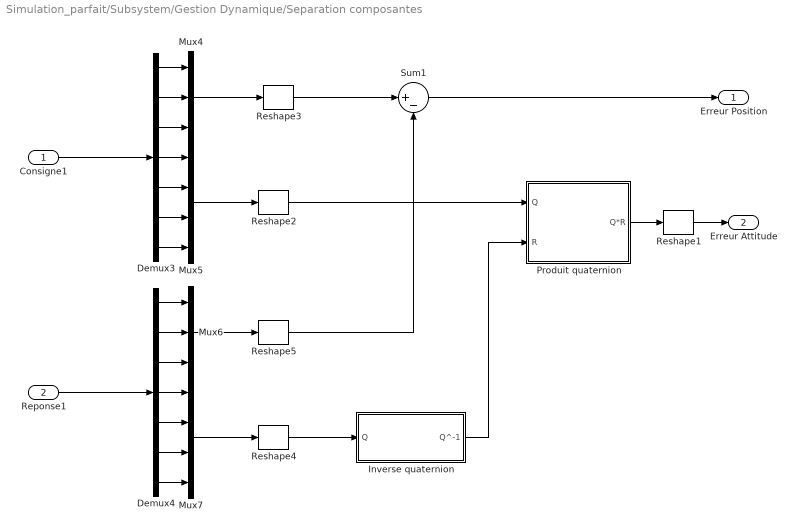
== system Simulation_parfait/Subsystem/Gestion Dynamique/Separation composantes ==
  Consigne1 : Inport  Port=1  LatchInput=off
  Reponse1 : Inport  Port=2  LatchInput=off
  Demux3 : Demux  Outputs=7
  Demux4 : Demux  Outputs=7
  Inverse quaternion : Subsystem
  Mux4 : Mux  Inputs=3
  Mux5 : Mux
  Mux6 : Mux  Inputs=3
  Mux7 : Mux
  Produit quaternion : Subsystem
  Reshape{1..5} (5 alike) : simulink/Math Operations/Reshape  OutputDimensionality=1-D array  OutputDimensions=[1,1]
  Sum1 : Sum  Inputs=|+-
  Erreur Position : Outport
      settings: BusObject=perturbations
  Erreur Attitude : Outport  Port=2
      settings: BusObject=perturbations
  wires:
  Consigne1/1 -> Demux3/1
  Demux3/4 -> Mux5/1
  Demux3/5 -> Mux5/2
  Demux3/6 -> Mux5/3
  Demux3/7 -> Mux5/4
  Demux3/3 -> Mux4/3
  Demux3/2 -> Mux4/2
  Demux3/1 -> Mux4/1
  Mux5/1 -> Reshape2/1
  Mux4/1 -> Reshape3/1
  Demux4/4 -> Mux7/1
  Demux4/5 -> Mux7/2
  Demux4/6 -> Mux7/3
  Demux4/7 -> Mux7/4
  Demux4/3 -> Mux6/3
  Demux4/2 -> Mux6/2
  Demux4/1 -> Mux6/1
  Reponse1/1 -> Demux4/1
  Mux7/1 -> Reshape4/1
  Mux6/1 -> Reshape5/1
  Reshape3/1 -> Sum1/1
  Reshape5/1 -> Sum1/2
  Sum1/1 -> Erreur Position/1
  Reshape4/1 -> Inverse quaternion/1(Q)
  Reshape2/1 -> Produit quaternion/1(Q)
  Inverse quaternion/1(Q^-1) -> Produit quaternion/2(R)
  Produit quaternion/1(Q*R) -> Reshape1/1
  Reshape1/1 -> Erreur Attitude/1

== system Simulation_parfait/Subsystem/Gestion Dynamique/Separation composantes1 ==
  Entree : Inport  Port=1  LatchInput=off
  Demux1 : Demux  Outputs=7
  Mux : Mux  Inputs=3
  Mux1 : Mux
  Reshape : simulink/Math Operations/Reshape  OutputDimensionality=1-D array  OutputDimensions=[1,1]
  Reshape1 : simulink/Math Operations/Reshape  OutputDimensionality=1-D array  OutputDimensions=[1,1]
  Position : Outport
      settings: BusObject=perturbations
  Orientation : Outport  Port=2
      settings: BusObject=perturbations
  wires:
  Entree/1 -> Demux1/1
  Demux1/4 -> Mux1/1
  Demux1/5 -> Mux1/2
  Demux1/6 -> Mux1/3
  Demux1/7 -> Mux1/4
  Demux1/3 -> Mux/3
  Demux1/2 -> Mux/2
  Demux1/1 -> Mux/1
  Mux1/1 -> Reshape/1
  Mux/1 -> Reshape1/1
  Reshape/1 -> Orientation/1
  Reshape1/1 -> Position/1

== system Simulation_parfait/Subsystem/Gestion Dynamique/Sommation ordres ==
  Ordres position : Inport  Port=1  LatchInput=off
  Ordres orientation : Inport  Port=2  LatchInput=off
  Sum : Sum
  Ordres : Outport
      settings: BusObject=perturbations
  wires:
  Ordres orientation/1 -> Sum/2
  Sum/1 -> Ordres/1
  Ordres position/1 -> Sum/1

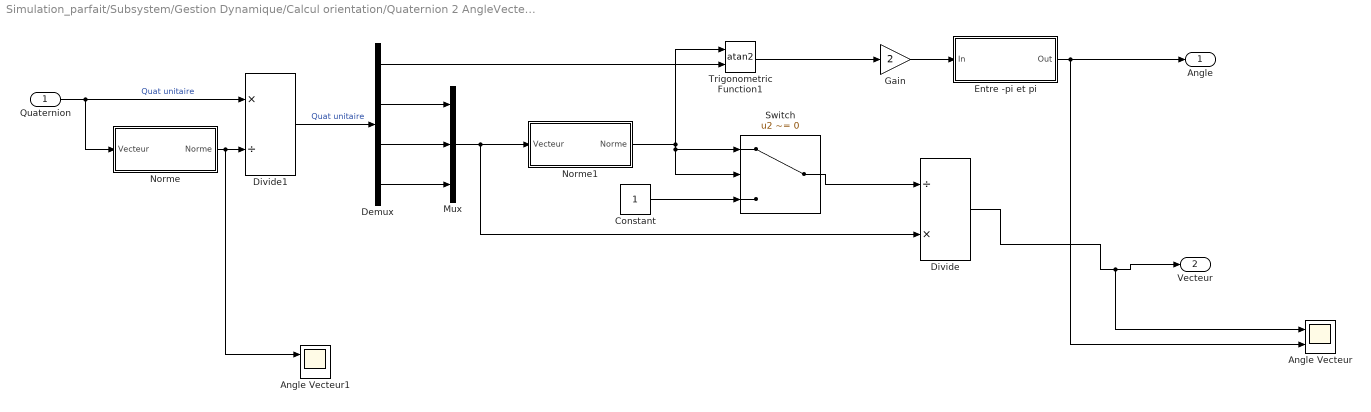
== system Simulation_parfait/Subsystem/Gestion Dynamique/Calcul orientation/Quaternion 2 AngleVecteur ==
  Quaternion : Inport  Port=1  LatchInput=off
  Angle Vecteur : Scope  NumInputPorts=2
      settings: YMin=-5~-5  YMax=5~5  SaveName=ScopeData10
  Angle Vecteur1 : Scope  NumInputPorts=2
      settings: YMin=0.007~-5  YMax=0.01025~5  SaveName=ScopeData17
  Constant : Constant
  Demux : Demux
  Divide : Product  Inputs=/*  OutScaling=2^-10
  Divide1 : Product  Inputs=*/  OutScaling=2^-10
  Entre -pi et pi : Subsystem  mask{ordre=2}
  Gain : Gain  Gain=2
  Mux : Mux  Inputs=3
  Norme : Subsystem  mask{ordre=2}
      mask Display: text(0.3,0.5,strcat('Norme',get_param(gcb, 'ordre')));
  Norme1 : Subsystem  mask{ordre=2}
      mask Display: text(0.3,0.5,strcat('Norme',get_param(gcb, 'ordre')));
  Switch : Switch  Criteria=u2 ~= 0
  Trigonometric Function1 : Trigonometry  Operator=atan2
  Angle : Outport
  Vecteur : Outport  Port=2
  wires:
  Quaternion/1 -> Divide1/1, Norme/1(Vecteur)  "Quat unitaire"
  Trigonometric Function1/1 -> Gain/1
  Mux/1 -> Norme1/1(Vecteur), Divide/2
  Demux/2 -> Mux/1
  Demux/3 -> Mux/2
  Demux/4 -> Mux/3
  Norme1/1(Norme) -> Trigonometric Function1/1, Switch/2, Switch/1
  Demux/1 -> Trigonometric Function1/2
  Switch/1 -> Divide/1
  Constant/1 -> Switch/3
  Entre -pi et pi/1(Out) -> Angle/1, Angle Vecteur/2
  Gain/1 -> Entre -pi et pi/1(In)
  Divide/1 -> Vecteur/1, Angle Vecteur/1
  Divide1/1 -> Demux/1  "Quat unitaire"
  Norme/1(Norme) -> Divide1/2, Angle Vecteur1/1

== system Simulation_parfait/Subsystem/Gestion Dynamique/Separation composantes/Inverse quaternion ==
  Q : Inport  Port=1  LatchInput=off
  Gain : Gain  Gain=[1 -1 -1 -1]
  Q^-1 : Outport
  wires:
  Q/1 -> Gain/1
  Gain/1 -> Q^-1/1

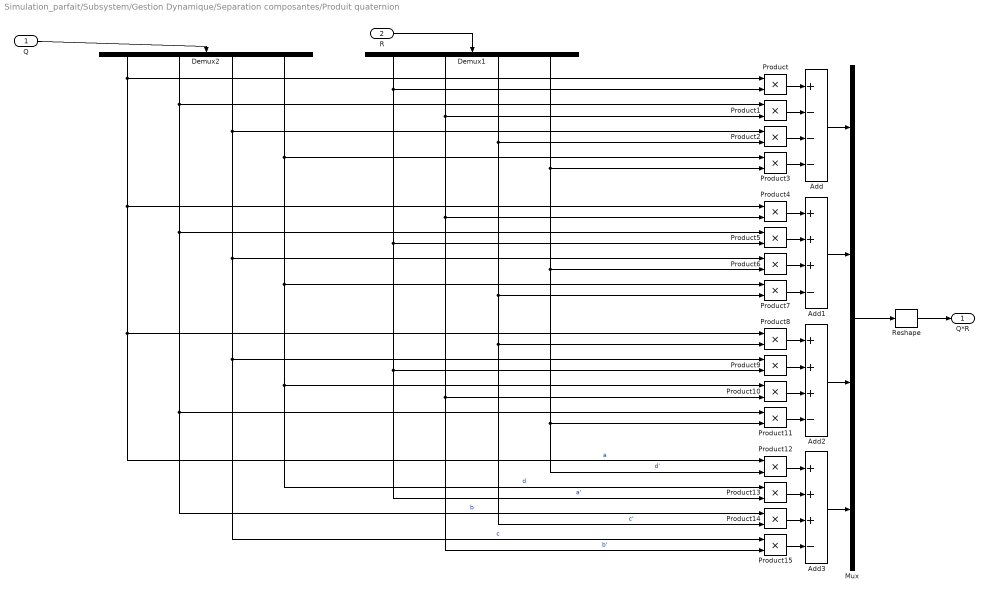
== system Simulation_parfait/Subsystem/Gestion Dynamique/Separation composantes/Produit quaternion ==
  Q : Inport  Port=1  LatchInput=off
  R : Inport  Port=2  LatchInput=off
  Add : Sum  Inputs=+---  OutScaling=2^-10
  Add1 : Sum  Inputs=+++-  OutScaling=2^-10
  Add2 : Sum  Inputs=+++-  OutScaling=2^-10
  Add3 : Sum  Inputs=+++-  OutScaling=2^-10
  Demux1 : Demux  Orientation=down
  Demux2 : Demux  Orientation=down
  Mux : Mux
  Product{,1..15} (16 alike) : Product  RndMeth=Zero
  Reshape : simulink/Math Operations/Reshape  OutputDimensionality=1-D array  OutputDimensions=[1,1]
  Q*R : Outport
  wires:
  R/1 -> Demux1/1
  Q/1 -> Demux2/1
  Mux/1 -> Reshape/1
  Reshape/1 -> Q*R/1
  Demux2/1 -> Product/1, Product4/1, Product8/1, Product12/1  "a"
  Add/1 -> Mux/1
  Add1/1 -> Mux/2
  Add2/1 -> Mux/3
  Add3/1 -> Mux/4
  Product3/1 -> Add/4
  Product2/1 -> Add/3
  Product1/1 -> Add/2
  Product/1 -> Add/1
  Product7/1 -> Add1/4
  Product6/1 -> Add1/3
  Product5/1 -> Add1/2
  Product4/1 -> Add1/1
  Product11/1 -> Add2/4
  Product10/1 -> Add2/3
  Product9/1 -> Add2/2
  Product8/1 -> Add2/1
  Product15/1 -> Add3/4
  Product14/1 -> Add3/3
  Product13/1 -> Add3/2
  Product12/1 -> Add3/1
  Demux2/2 -> Product1/1, Product5/1, Product11/1, Product14/1  "b"
  Demux2/3 -> Product2/1, Product6/1, Product9/1, Product15/1  "c"
  Demux2/4 -> Product3/1, Product7/1, Product10/1, Product13/1  "d"
  Demux1/1 -> Product/2, Product5/2, Product9/2, Product13/2  "a'"
  Demux1/2 -> Product1/2, Product4/2, Product10/2, Product15/2  "b'"
  Demux1/3 -> Product2/2, Product7/2, Product8/2, Product14/2  "c'"
  Demux1/4 -> Product3/2, Product6/2, Product11/2, Product12/2  "d'"

== system Simulation_parfait/Subsystem/Gestion Dynamique/Calcul orientation/Quaternion 2 AngleVecteur/Entre -pi et pi ==
  In : Inport  Port=1  LatchInput=off
  Constant1 : Constant  Value=pi
  Constant2 : Constant  Value=2*pi
  Constant3 : Constant  Value=pi
  Math Function3 : Math  Operator=mod  SaturateOnIntegerOverflow=on
  Subtract : Sum  OutScaling=2^-10
  Subtract1 : Sum  Inputs=+-  OutScaling=2^-10
  Out : Outport
  wires:
  Subtract/1 -> Math Function3/1
  Constant2/1 -> Math Function3/2
  In/1 -> Subtract/1
  Constant1/1 -> Subtract/2
  Math Function3/1 -> Subtract1/1
  Constant3/1 -> Subtract1/2
  Subtract1/1 -> Out/1

== system Simulation_parfait/Subsystem/Gestion Dynamique/Calcul orientation/Quaternion 2 AngleVecteur/Norme ==
  Vecteur : Inport  Port=1  LatchInput=off
  Constant1 : Constant  Value=ordre
  Math Function : Math  Operator=pow  SaturateOnIntegerOverflow=on
  Math Function1 : Math  Operator=reciprocal  SaturateOnIntegerOverflow=on
  Math Function2 : Math  Operator=pow  SaturateOnIntegerOverflow=on
  Sum of Elements : Sum  Inputs=+  OutScaling=2^-10
  Norme : Outport
  wires:
  Math Function/1 -> Sum of Elements/1
  Vecteur/1 -> Math Function/1
  Constant1/1 -> Math Function/2, Math Function1/1
  Math Function1/1 -> Math Function2/2
  Sum of Elements/1 -> Math Function2/1
  Math Function2/1 -> Norme/1

== system Simulation_parfait/Subsystem/Gestion Dynamique/Calcul orientation/Quaternion 2 AngleVecteur/Norme1 ==
  Vecteur : Inport  Port=1  LatchInput=off
  Constant1 : Constant  Value=ordre
  Math Function : Math  Operator=pow  SaturateOnIntegerOverflow=on
  Math Function1 : Math  Operator=reciprocal  SaturateOnIntegerOverflow=on
  Math Function2 : Math  Operator=pow  SaturateOnIntegerOverflow=on
  Sum of Elements : Sum  Inputs=+  OutScaling=2^-10
  Norme : Outport
  wires:
  Math Function/1 -> Sum of Elements/1
  Vecteur/1 -> Math Function/1
  Constant1/1 -> Math Function/2, Math Function1/1
  Math Function1/1 -> Math Function2/2
  Sum of Elements/1 -> Math Function2/1
  Math Function2/1 -> Norme/1
